simulink model "topController"  (R2013b)
settings: Solver=FixedStepDiscrete  StartTime=0.0  StopTime=10.0  FixedStep=0.01  RelTol=1e-3
settings Model: Creator=Raj  LastModifiedBy=Raj
settings OptimizationCC: OptimizeModelRefInitCode=on  LifeSpan=1
settings HardwareCC: ProdLargestAtomicInteger=Long  ProdLargestAtomicFloat=Double  ProdEndianess=LittleEndian  ProdHWDeviceType=ARM Compatible->ARM Cortex
settings RTWCC: SystemTargetFile=ert.tlc  GenCodeOnly=on  TemplateMakefile=ert_default_tmf  Description=Embedded Coder  ProcessScript=ert_make_rtw_hook  Toolchain=GNU Tools for ARM Embedded Processors
settings CodeAppCC: IgnoreCustomStorageClasses=off
settings ERTTargetCC: CodeReplacementLibrary=ANSI_C  IncludeMdlTerminateFcn=off  ERTCustomFileTemplate=example_file_process.tlc

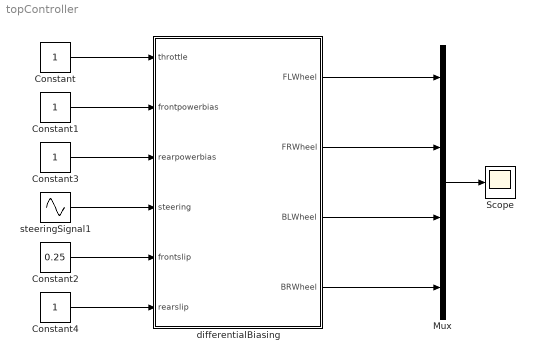
== system topController ==
  Constant{,1,3..4} (4 alike) : Constant
  Constant2 : Constant  Value=0.25
  Mux : Mux
  Scope : Scope
  differentialBiasing : Subsystem
  steeringSignal1 : Sin  Frequency=5  SampleTime=0
  wires:
  differentialBiasing/4(BRWheel) -> Mux/4
  differentialBiasing/3(BLWheel) -> Mux/3
  differentialBiasing/1(FLWheel) -> Mux/1
  differentialBiasing/2(FRWheel) -> Mux/2
  Mux/1 -> Scope/1
  Constant/1 -> differentialBiasing/1(throttle)
  Constant1/1 -> differentialBiasing/2(frontpowerbias)
  Constant3/1 -> differentialBiasing/3(rearpowerbias)
  Constant2/1 -> differentialBiasing/5(frontslip)
  Constant4/1 -> differentialBiasing/6(rearslip)
  steeringSignal1/1 -> differentialBiasing/4(steering)

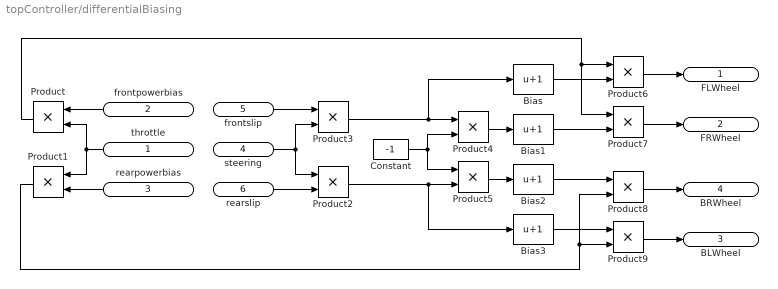
== system topController/differentialBiasing ==
  throttle : Inport
  frontpowerbias : Inport  Port=2
  rearpowerbias : Inport  Port=3
  steering : Inport  Port=4
  frontslip : Inport  Port=5
  rearslip : Inport  Port=6
  Bias{,1..3} (4 alike) : Bias  Bias=1
  Constant : Constant  Value=-1
  Product{,1..9} (10 alike) : Product
  FLWheel : Outport
  FRWheel : Outport  Port=2
  BLWheel : Outport  Port=3
  BRWheel : Outport  Port=4
  wires:
  frontpowerbias/1 -> Product/1
  rearpowerbias/1 -> Product1/2
  rearslip/1 -> Product2/2
  frontslip/1 -> Product3/1
  throttle/1 -> Product1/1, Product/2
  Constant/1 -> Product5/1, Product4/2
  Product3/1 -> Bias/1, Product4/1
  Bias1/1 -> Product7/2
  Product5/1 -> Bias2/1
  Product4/1 -> Bias1/1
  Bias2/1 -> Product8/1
  Bias/1 -> Product6/2
  Product/1 -> Product6/1, Product7/1
  Bias3/1 -> Product9/1
  Product2/1 -> Product5/2, Bias3/1
  Product1/1 -> Product9/2, Product8/2
  steering/1 -> Product2/1, Product3/2
  Product9/1 -> BLWheel/1
  Product8/1 -> BRWheel/1
  Product7/1 -> FRWheel/1
  Product6/1 -> FLWheel/1
